simulink model "part2"  (R2019b)
settings: Solver=FixedStepAuto  StartTime=0.0  StopTime=1000  FixedStep=0.1  RelTol=1e-3
values from neighbouring files (symbols this model uses):
  A_w = [zeros(3) eye(3) ... (first row only)    [initObs.m]
  B_pseudo = inv(W)*B_u'*inv(B_u*inv(W)*B_u' + epsilon.*eye(3))    [init_thrustAloc.m]
  C_w = [zeros(3) eye(3)]    [initObs.m]
  constant_dp = 0    [pick_sp.m]
  corner_test = 0    [pick_sp.m]
  corners = [0,0,0;50,0,0;50,-50,0;50,-50,-pi/4;0,-50,-pi/4;0,0,0]    [pick_sp.m]
  curr_mean_dir = curr_mean_dir + 10    (= 10)    [capabilitytest.m]    (also in pick_sp.m = 270)
  curr_mean_vel = 0.2    [pick_sp.m]
  D = diag([2.6486e+05,8.8164e+05,3.3774e+08])    [init.m]    (also in initObs.m = [2.648*10^5 0 0)
  Delta_stack = zeros(15,3,360)    [init_kalman.m]
  Gamma_stack = zeros(15,6,360)    [init_kalman.m]
  H = [Cw, eye(3),zeros(3,6)]    [init_kalman.m]
  K1 = [-2*(zeta_ni_nop - zeta_i_nop)*(omega_ci_nop/omega_p)*eye(3) ... (first row only)    [initObs.m]
  K2 = diag([omega_ci_nop omega_ci_nop omega_ci_nop])    [initObs.m]
  K3 = 0.1*K4    [initObs.m]
  K4 = diag([0.1 0.1 0.01])    [initObs.m]
  Kd = [1e+07,1e+07,2.01e+08]    [tune.m]
  Ki = [2e+02,2e+02,1e+02]    [tune.m]
  Kp = [1e+05,5e+05,1e+07]    [tune.m]
  M = [6.8177e+06,0,0;0,7.8784e+06,-2.5955e+06;0,-2.5955e+06,3.57e+09]    [init.m]    (also in initObs.m = [ 6.8177*10^6 0 0)
  observer_on = 1    [pick_sp.m]
  Phi_stack = zeros(15,15,360)    [init_kalman.m]
  Q = diag([Q1 Q2])    [init_kalman.m]
  R_KF = diag([0 0 0])    [init_kalman.m]
  ref_model_on = 1    [pick_sp.m]
  setpoint = [0,0,0]    [pick_sp.m]
  T_b = diag([1000 1000 1000])    [initObs.m]
  thrusters =     [thrusters_sup.mat]
  use_kalman = 1    [pick_sp.m]
  vessel =     [thrusters_sup.mat]
  w_n = [0.08,0.04,0.03]    [tune.m]
  wave_mean_dir = wave_mean_dir + (10*pi/180)    (= 0.174532925199)    [capabilitytest.m]    (also in pick_sp.m = 225)
  wave_peak_T = 13    [pick_sp.m]
  wind_mean_dir = wind_mean_dir + (10*pi/180)    (= 0.174532925199)    [capabilitytest.m]    (also in pick_sp.m = 180)
  wind_mean_vel = 15    [pick_sp.m]
  zeta = 1    [tune.m]
undefined symbols (not defined in the file or in its folder): Hoerner, magnitude
libraries: marine_gnc x13, simulink x4, cstblocks x4, marine_hydro x2
(part 1 of 2)
settings Model: Creator=jonbjor  LastModifiedBy=Elias
settings DataIOCC: ReturnWorkspaceOutputs=off
settings DebuggingCC: ArithmeticOperatorsInVariantConditions=warning
settings SFSimCC: SimUseLocalCustomCode=off  CustomCodeUndefinedFunction=UseInterfaceOnly
settings RTWCC: RTWUseLocalCustomCode=off

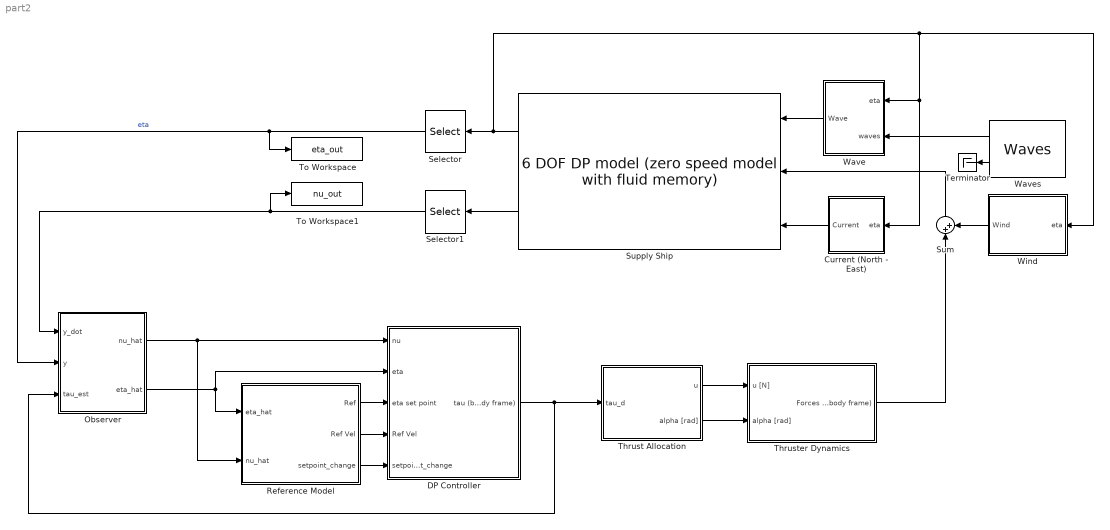
== system part2 ==
  Current (North - East) : Subsystem
  DP Controller : Subsystem
  Observer : Subsystem
  Reference Model : Subsystem
  Selector : Selector  InputPortWidth=6  IndexOptions=Index vector (dialog)  Indices=[1 2 6]  OutputSizes=1
  Selector1 : Selector  InputPortWidth=6  IndexOptions=Index vector (dialog)  Indices=[1 2 6]  OutputSizes=1
  Sum : Sum  Inputs=|++
  Supply Ship : marine_hydro/Hydro Library/6 DOF DP model  (zero speed model with fluid memory)  ABC=vesselABC  rho=1025  Axc=0.9*vessel.main.T*vessel.main.B  Ayc=0.9*vessel.main.T*vessel.main.Lpp  CX=1  CY_2D=Hoerner(vessel.main.B,vessel.main.T)  Bv=vessel.Bv  mask(6 DOF zero speed model){}
      link override "Integrator1 ": InitialCondition=nu0
      link override Integrator2: InitialCondition=eta0
      settings: SourceProductName=MSS Hydro
      mask Display:
      | image('supply.jpg');
      | color('white'); port_label('output', 1, 'eta')
      | color('white'); port_label('output', 2, 'nu')
      | color('white'); port_label('input', 1, 'tau_wave')
      | color('white'); port_label('input', 2, 'tau')
      | color('white'); port_label('input', 3, 'nu_c')
  Terminator : Terminator
  Thrust Allocation : Subsystem
  Thruster Dynamics : Subsystem  mask{thrusterfault=off}
      mask prompts: thrusterfault "Fault on thruster #2 and #5?"
  To Workspace : ToWorkspace  VariableName=eta_out  SampleTime=-1
  To Workspace1 : ToWorkspace  VariableName=nu_out  SampleTime=-1
  Wave : Subsystem  mask{waveforces=off}
      mask prompts: waveforces "Waveforces enabled"
  Waves : marine_gnc/Environment/Waves/Waves  spectrum_type=ITTC  disp_flag=on  plot_spectrum=off  plot_realization=off  hs=wave_height  omega_peak=2*pi/wave_peak_T  psi_mean=wave_mean_dir*pi/180  gamma=-1  spread=2  depth=inf  nfreq=100  ndir=10  energylim=0.005  freq_cutoff=3  dir_cutoff=0  rand_seed=1234  rand_freq=off  rand_dir=off  Zeta_a=0  Omega=0  Phase=0  Wavenum=0  Psi=0
      settings: SourceProductName=MSS GNC
  Wind : Subsystem
  wires:
  Supply Ship/2 -> Selector1/1
  Supply Ship/1 -> Wind/1("eta "), Current (North - East)/1(eta), Wave/1(eta), Selector/1
  Waves/1 -> Wave/2(waves)
  Waves/2 -> Terminator/1
  Selector1/1 -> To Workspace1/1, Observer/1(y_dot)
  Observer/1(nu_hat) -> Reference Model/2(nu_hat), DP Controller/1(nu)
  Sum/1 -> Supply Ship/2
  Selector/1 -> To Workspace/1, Observer/2(y)  "eta"
  Reference Model/1("Ref ") -> DP Controller/3(eta set point)
  Observer/2(eta_hat) -> Reference Model/1(eta_hat), DP Controller/2(eta)
  Reference Model/2("Ref Vel ") -> DP Controller/4("Ref Vel ")
  Current (North - East)/1(Current) -> Supply Ship/3
  Wave/1(Wave) -> Supply Ship/1
  Wind/1(Wind) -> Sum/2
  Thrust Allocation/2(alpha [rad]) -> Thruster Dynamics/2(alpha [rad])
  Thruster Dynamics/1("Forces (body frame) ") -> Sum/1
  Thrust Allocation/1("u ") -> Thruster Dynamics/1(u [N])
  DP Controller/1(tau (body frame)) -> Thrust Allocation/1(tau_d), Observer/3(tau_est)
  Reference Model/3(setpoint_change) -> DP Controller/5(setpoint_change)

== system part2/Current (North - East) ==
  eta : Inport
  "Angle variation " : Subsystem
  Constant : Constant  Value=curr_mean_vel
  Constant2 : Constant  Value=curr_mean_dir
  North-East current : marine_gnc/Environment/Current/North-East current  SystemSampleTime=-1  Latency=0  AutoFrameSizeCalculation=off
      settings: SourceProductName=MSS GNC
  "RFC " : Subsystem
  Velocity variation : Subsystem
  Current : Outport  VectorParamsAs1DForOutWhenUnconnected=off
  wires:
  Constant/1 -> Velocity variation/1(Mean Vel)
  eta/1 -> "RFC "/1(eta)
  North-East current/1 -> "RFC "/2("Current (NED) ")
  "RFC "/1("Current (Body) ") -> Current/1
  Constant2/1 -> "Angle variation "/1(Mean Dir)
  "Angle variation "/1(Current Dir) -> North-East current/1
  Velocity variation/1(Current Vel) -> North-East current/2

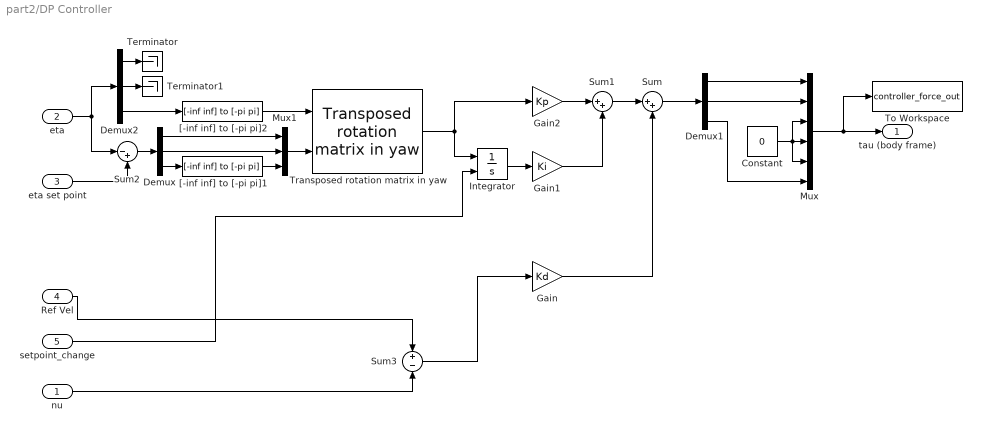
== system part2/DP Controller ==
  nu : Inport  PortDimensions=3
  eta : Inport  Port=2  PortDimensions=3
  eta set point : Inport  Port=3
  "Ref Vel " : Inport  Port=4
  setpoint_change : Inport  Port=5
  Constant : Constant  Value=0
  Demux : Demux  Outputs=3
  Demux1 : Demux  Outputs=3
  Demux2 : Demux  Outputs=3
  Gain : Gain  Gain=Kd
  Gain1 : Gain  Gain=Ki
  Gain2 : Gain  Gain=Kp
  Integrator : Integrator  ExternalReset=level hold
  Mux : Mux  Inputs=6
  Mux1 : Mux  Inputs=3
  Sum : Sum  Inputs=|++
  Sum1 : Sum  Inputs=|++
  Sum2 : Sum  Inputs=|-+
  Sum3 : Sum  Inputs=+|-
  Terminator : Terminator
  Terminator1 : Terminator
  To Workspace : ToWorkspace  VariableName=controller_force_out  SampleTime=-1
  Transposed rotation matrix in yaw : marine_gnc/Models/ Kinematics/Transposed rotation  matrix in yaw
      settings: SourceProductName=MSS GNC
  "[-inf inf] to [-pi pi]1" : marine_gnc/Utilities/Math Operations/[-inf inf] to [-pi pi]
      settings: SourceProductName=MSS GNC
  "[-inf inf] to [-pi pi]2" : marine_gnc/Utilities/Math Operations/[-inf inf] to [-pi pi]
      settings: SourceProductName=MSS GNC
  tau (body frame) : Outport  VectorParamsAs1DForOutWhenUnconnected=off
  wires:
  Demux2/2 -> Terminator1/1
  Demux/3 -> "[-inf inf] to [-pi pi]1"/1
  Sum2/1 -> Demux/1
  Demux1/1 -> Mux/1
  "[-inf inf] to [-pi pi]2"/1 -> Transposed rotation matrix in yaw/1
  "[-inf inf] to [-pi pi]1"/1 -> Mux1/3
  Mux/1 -> To Workspace/1, tau (body frame)/1
  Demux/1 -> Mux1/1
  Demux1/2 -> Mux/2
  Demux2/3 -> "[-inf inf] to [-pi pi]2"/1
  Constant/1 -> Mux/5, Mux/3, Mux/4
  Mux1/1 -> Transposed rotation matrix in yaw/2
  Integrator/1 -> Gain1/1
  eta/1 -> Demux2/1, Sum2/1
  Gain2/1 -> Sum1/1
  Gain1/1 -> Sum1/2
  Demux2/1 -> Terminator/1
  Demux/2 -> Mux1/2
  Demux1/3 -> Mux/6
  Sum/1 -> Demux1/1
  Sum1/1 -> Sum/1
  Gain/1 -> Sum/2
  eta set point/1 -> Sum2/2
  Transposed rotation matrix in yaw/1 -> Integrator/1, Gain2/1
  nu/1 -> Sum3/2
  Sum3/1 -> Gain/1
  "Ref Vel "/1 -> Sum3/1
  setpoint_change/1 -> Integrator/2

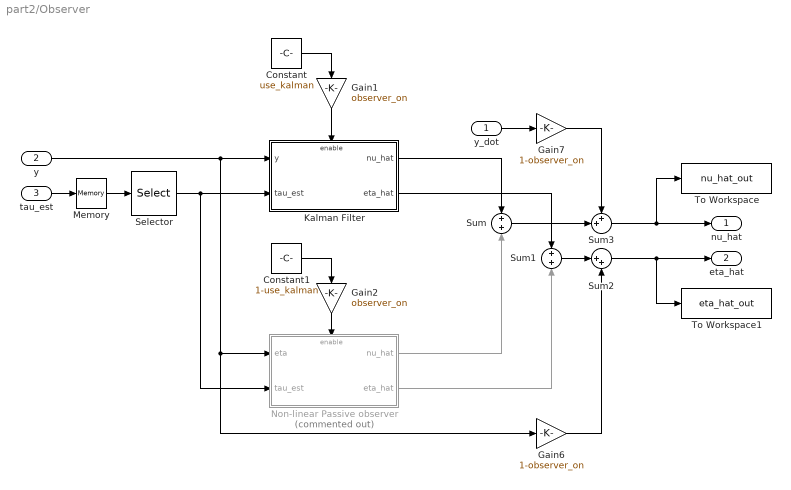
== system part2/Observer ==
  y_dot : Inport
  y : Inport  Port=2
  tau_est : Inport  Port=3
  Constant : Constant  Value=use_kalman
  Constant1 : Constant  Value=1-use_kalman
  Gain1 : Gain  Gain=observer_on
  Gain2 : Gain  Gain=observer_on
  Gain6 : Gain  Gain=1-observer_on
  Gain7 : Gain  Gain=1-observer_on
  "Kalman Filter " : Subsystem
  Memory : Memory
  Non-linear Passive observer : Subsystem  Commented=on
  Selector : Selector  InputPortWidth=6  IndexOptions=Index vector (dialog)  Indices=[1 2 6]  OutputSizes=1
  Sum : Sum  Inputs=+|+
  Sum1 : Sum  Inputs=+|+
  Sum2 : Sum  Inputs=|++
  Sum3 : Sum  Inputs=++|
  To Workspace : ToWorkspace  VariableName=nu_hat_out  SampleTime=-1
  To Workspace1 : ToWorkspace  VariableName=eta_hat_out  SampleTime=-1
  nu_hat : Outport  VectorParamsAs1DForOutWhenUnconnected=off
  eta_hat : Outport  Port=2  VectorParamsAs1DForOutWhenUnconnected=off
  wires:
  Gain6/1 -> Sum2/2
  y_dot/1 -> Gain7/1
  Gain7/1 -> Sum3/1
  Sum3/1 -> To Workspace/1, nu_hat/1
  Sum2/1 -> To Workspace1/1, eta_hat/1
  y/1 -> "Kalman Filter "/1(y), Non-linear Passive observer/1(eta), Gain6/1
  tau_est/1 -> Memory/1
  "Kalman Filter "/1(nu_hat) -> Sum/1
  "Kalman Filter "/2(eta_hat) -> Sum1/1
  Non-linear Passive observer/1(nu_hat) -> Sum/2
  Non-linear Passive observer/2(eta_hat) -> Sum1/2
  Sum/1 -> Sum3/2
  Sum1/1 -> Sum2/1
  Constant/1 -> Gain1/1
  Gain1/1 -> "Kalman Filter "/Enable
  Constant1/1 -> Gain2/1
  Gain2/1 -> Non-linear Passive observer/Enable
  Selector/1 -> Non-linear Passive observer/2(tau_est), "Kalman Filter "/2(tau_est)
  Memory/1 -> Selector/1

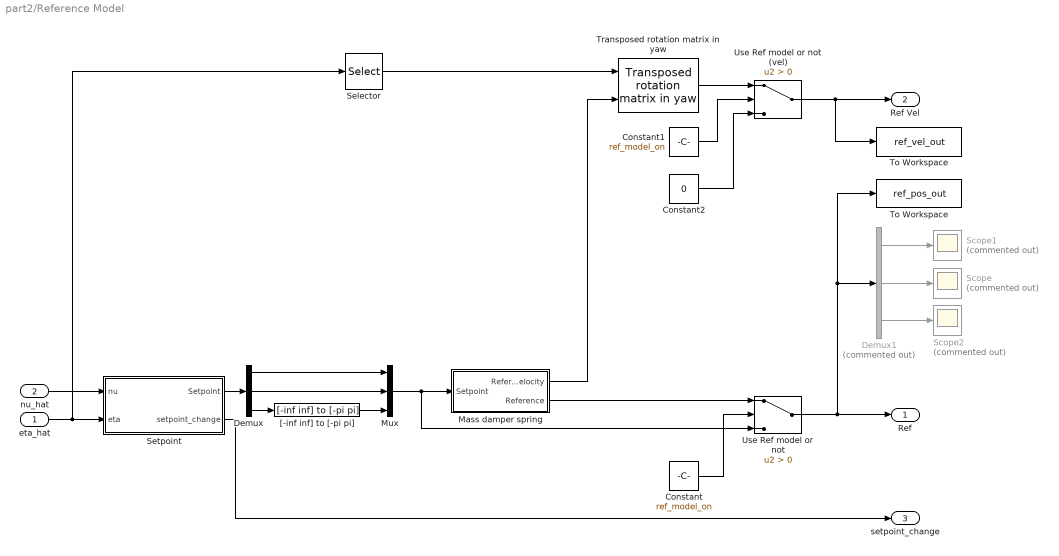
== system part2/Reference Model ==
  eta_hat : Inport
  nu_hat : Inport  Port=2
  Constant : Constant  Value=ref_model_on
  Constant1 : Constant  Value=ref_model_on
  Constant2 : Constant  Value=0
  Demux : Demux  Outputs=3
  Demux1 : Demux  Commented=on  Outputs=3
  Mass damper spring : Subsystem
  Mux : Mux  Inputs=3
  Scope : Scope  Commented=on
  Scope1 : Scope  Commented=on
  Scope2 : Scope  Commented=on
  Selector : Selector  InputPortWidth=3  IndexOptions=Index vector (dialog)  Indices=[3]  OutputSizes=1
  "Setpoint " : Subsystem
  To Workspace : ToWorkspace  VariableName=ref_vel_out  SampleTime=-1
  "To Workspace " : ToWorkspace  VariableName=ref_pos_out  SampleTime=-1
  Transposed rotation matrix in yaw : marine_gnc/Models/ Kinematics/Transposed rotation  matrix in yaw
      settings: SourceProductName=MSS GNC
  Use Ref model or not : Switch  Criteria=u2 > Threshold
  "Use Ref model or not (vel) " : Switch  Criteria=u2 > Threshold
  "[-inf inf] to [-pi pi]" : marine_gnc/Utilities/Math Operations/[-inf inf] to [-pi pi]
      settings: SourceProductName=MSS GNC
  "Ref " : Outport  VectorParamsAs1DForOutWhenUnconnected=off
  "Ref Vel " : Outport  Port=2  VectorParamsAs1DForOutWhenUnconnected=off
  setpoint_change : Outport  Port=3
  wires:
  Mass damper spring/2("Reference ") -> Use Ref model or not/1
  Use Ref model or not/1 -> "Ref "/1, "To Workspace "/1, Demux1/1
  Mass damper spring/1("Reference Velocity ") -> Transposed rotation matrix in yaw/2
  Mux/1 -> Use Ref model or not/3, Mass damper spring/1("Setpoint ")
  Demux1/2 -> Scope/1
  Demux/3 -> "[-inf inf] to [-pi pi]"/1
  "[-inf inf] to [-pi pi]"/1 -> Mux/3
  Demux1/3 -> Scope2/1
  Demux1/1 -> Scope1/1
  "Setpoint "/1("Setpoint ") -> Demux/1
  Demux/1 -> Mux/1
  Demux/2 -> Mux/2
  Selector/1 -> Transposed rotation matrix in yaw/1
  eta_hat/1 -> Selector/1, "Setpoint "/2("eta ")
  nu_hat/1 -> "Setpoint "/1(nu)
  Constant/1 -> Use Ref model or not/2
  Transposed rotation matrix in yaw/1 -> "Use Ref model or not (vel) "/1
  Constant1/1 -> "Use Ref model or not (vel) "/2
  Constant2/1 -> "Use Ref model or not (vel) "/3
  "Use Ref model or not (vel) "/1 -> To Workspace/1, "Ref Vel "/1
  "Setpoint "/2(setpoint_change) -> setpoint_change/1

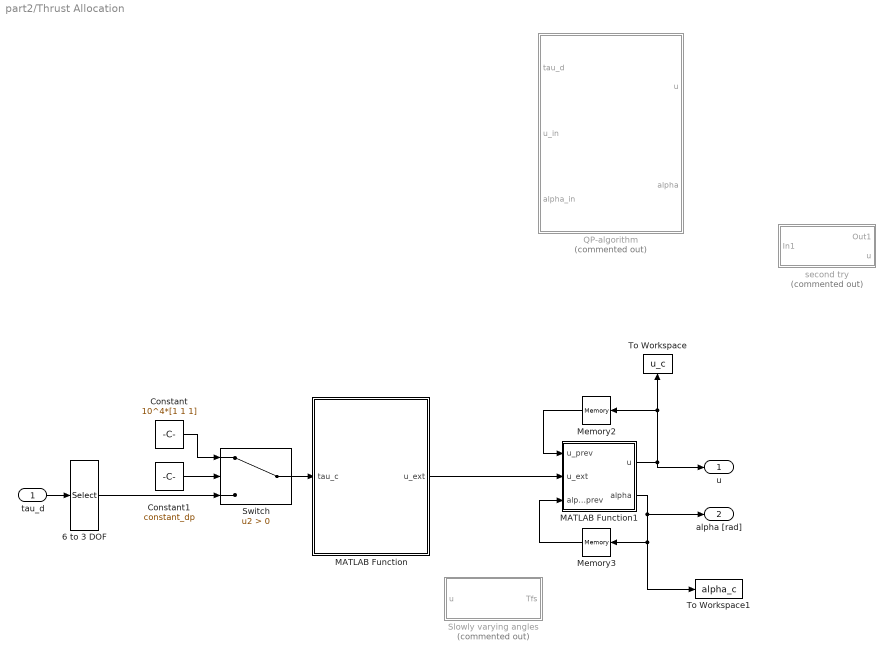
== system part2/Thrust Allocation ==
  tau_d : Inport
  6 to 3 DOF : Selector  InputPortWidth=6  IndexOptions=Index vector (dialog)  Indices=[1 2 6]  OutputSizes=1
  Constant : Constant  Value=10^4*[1 1 1]
  Constant1 : Constant  Value=constant_dp
  MATLAB Function : MATLAB Function  TreatAsAtomicUnit=on
  MATLAB Function1 : MATLAB Function  TreatAsAtomicUnit=on
  Memory2 : Memory
  Memory3 : Memory
  QP-algorithm : MATLAB Function  Commented=on  TreatAsAtomicUnit=on
  Slowly varying angles : Subsystem  Commented=on
  Switch : Switch  Criteria=u2 > Threshold
  To Workspace : ToWorkspace  VariableName=u_c  SampleTime=-1
  To Workspace1 : ToWorkspace  VariableName=alpha_c  SampleTime=-1
  second try : Subsystem  Commented=on
  "u " : Outport  VectorParamsAs1DForOutWhenUnconnected=off
  alpha [rad] : Outport  Port=2  VectorParamsAs1DForOutWhenUnconnected=off
  wires:
  tau_d/1 -> 6 to 3 DOF/1
  6 to 3 DOF/1 -> Switch/3
  MATLAB Function1/2(alpha) -> To Workspace1/1, Memory3/1, alpha [rad]/1
  MATLAB Function1/1(u) -> "u "/1, To Workspace/1, Memory2/1
  Memory3/1 -> MATLAB Function1/3(alpha_prev)
  Memory2/1 -> MATLAB Function1/1(u_prev)
  MATLAB Function/1(u_ext) -> MATLAB Function1/2(u_ext)
  Constant/1 -> Switch/1
  Switch/1 -> MATLAB Function/1(tau_c)
  Constant1/1 -> Switch/2

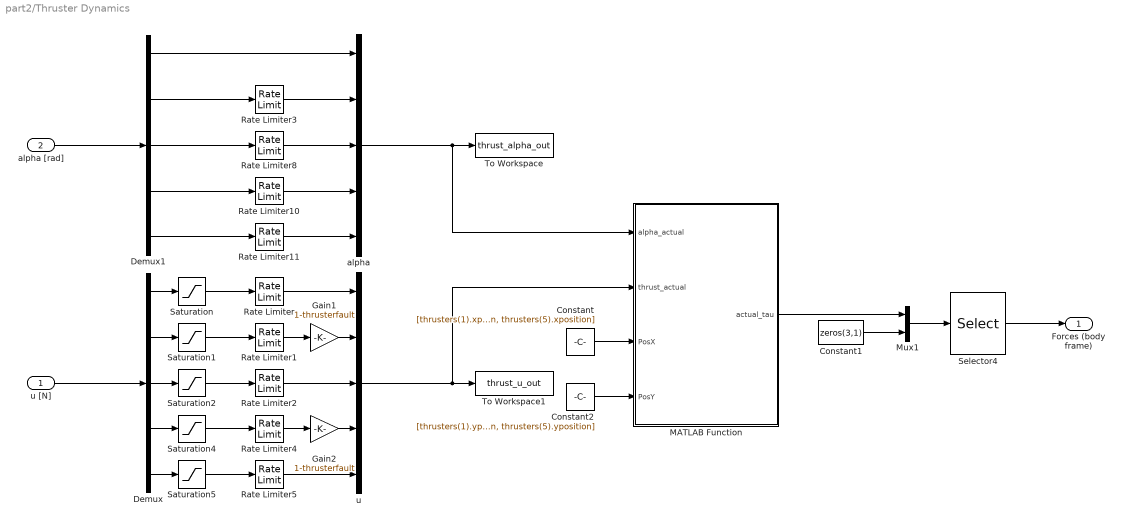
== system part2/Thruster Dynamics ==
  u [N] : Inport
  alpha [rad] : Inport  Port=2
  Constant : Constant  Value=[thrusters(1).xposition, thrusters(2).xposition, thrusters(3).xposition, thrusters(4).xposition, thrusters(5).xposition]
  Constant1 : Constant  Value=zeros(3,1)
  Constant2 : Constant  Value=[thrusters(1).yposition, thrusters(2).yposition, thrusters(3).yposition, thrusters(4).yposition, thrusters(5).yposition]
  Demux : Demux  Outputs=5
  Demux1 : Demux  Outputs=5
  Gain1 : Gain  Gain=1-thrusterfault
  Gain2 : Gain  Gain=1-thrusterfault
  MATLAB Function : MATLAB Function  TreatAsAtomicUnit=on
  Mux1 : Mux  Inputs=2
  Rate Limiter : RateLimiter  RisingSlewLimit=thrusters(1).rate  FallingSlewLimit=-thrusters(1).rate  SampleTimeMode=inherited
  Rate Limiter1 : RateLimiter  RisingSlewLimit=thrusters(2).rate  FallingSlewLimit=-thrusters(2).rate  SampleTimeMode=inherited
  Rate Limiter10 : RateLimiter  RisingSlewLimit=thrusters(4).rotationspeed  FallingSlewLimit=-thrusters(4).rotationspeed  SampleTimeMode=inherited
  Rate Limiter11 : RateLimiter  RisingSlewLimit=thrusters(5).rotationspeed  FallingSlewLimit=-thrusters(5).rotationspeed  SampleTimeMode=inherited
  Rate Limiter2 : RateLimiter  RisingSlewLimit=thrusters(3).rate  FallingSlewLimit=-thrusters(3).rate  SampleTimeMode=inherited
  Rate Limiter3 : RateLimiter  RisingSlewLimit=thrusters(2).rotationspeed  FallingSlewLimit=-thrusters(2).rotationspeed  SampleTimeMode=inherited
  Rate Limiter4 : RateLimiter  RisingSlewLimit=thrusters(4).rate  FallingSlewLimit=-thrusters(4).rate  SampleTimeMode=inherited
  Rate Limiter5 : RateLimiter  RisingSlewLimit=thrusters(5).rate  FallingSlewLimit=-thrusters(5).rate  SampleTimeMode=inherited
  Rate Limiter8 : RateLimiter  RisingSlewLimit=thrusters(3).rotationspeed  FallingSlewLimit=-thrusters(3).rotationspeed  SampleTimeMode=inherited
  Saturation : Saturate  UpperLimit=thrusters(1).thrust  LowerLimit=-thrusters(1).thrust
  Saturation1 : Saturate  UpperLimit=thrusters(2).thrust  LowerLimit=-thrusters(2).thrust
  Saturation2 : Saturate  UpperLimit=thrusters(3).thrust  LowerLimit=-thrusters(3).thrust
  Saturation4 : Saturate  UpperLimit=thrusters(4).thrust  LowerLimit=-thrusters(4).thrust
  Saturation5 : Saturate  UpperLimit=thrusters(5).thrust  LowerLimit=-thrusters(5).thrust
  Selector4 : Selector  InputPortWidth=6  IndexOptions=Index vector (dialog)  Indices=[1 2 4 5 6 3]  OutputSizes=1
  To Workspace : ToWorkspace  VariableName=thrust_alpha_out  SampleTime=-1
  To Workspace1 : ToWorkspace  VariableName=thrust_u_out  SampleTime=-1
  alpha : Mux  Inputs=5
  u : Mux  Inputs=5
  "Forces (body frame) " : Outport  VectorParamsAs1DForOutWhenUnconnected=off
  wires:
  Rate Limiter2/1 -> u/3
  Saturation/1 -> Rate Limiter/1
  Mux1/1 -> Selector4/1
  Constant1/1 -> Mux1/2
  Saturation4/1 -> Rate Limiter4/1
  Demux/2 -> Saturation1/1
  Saturation1/1 -> Rate Limiter1/1
  Demux/1 -> Saturation/1
  Demux/3 -> Saturation2/1
  Saturation2/1 -> Rate Limiter2/1
  Selector4/1 -> "Forces (body frame) "/1
  Gain1/1 -> u/2
  Rate Limiter1/1 -> Gain1/1
  Rate Limiter/1 -> u/1
  Rate Limiter4/1 -> Gain2/1
  Saturation5/1 -> Rate Limiter5/1
  Rate Limiter8/1 -> alpha/3
  u [N]/1 -> Demux/1
  alpha [rad]/1 -> Demux1/1
  Constant/1 -> MATLAB Function/3(PosX)
  Constant2/1 -> MATLAB Function/4(PosY)
  u/1 -> To Workspace1/1, MATLAB Function/2(thrust_actual)
  alpha/1 -> To Workspace/1, MATLAB Function/1(alpha_actual)
  MATLAB Function/1(actual_tau) -> Mux1/1
  Demux1/3 -> Rate Limiter8/1
  Rate Limiter10/1 -> alpha/4
  Demux1/4 -> Rate Limiter10/1
  Demux1/5 -> Rate Limiter11/1
  Rate Limiter11/1 -> alpha/5
  Demux1/2 -> Rate Limiter3/1
  Demux1/1 -> alpha/1
  Gain2/1 -> u/4
  Demux/4 -> Saturation4/1
  Demux/5 -> Saturation5/1
  Rate Limiter5/1 -> u/5
  Rate Limiter3/1 -> alpha/2

== system part2/Wave ==
  eta : Inport
  waves : Inport  Port=2
  Gain : Gain  Gain=waveforces
  Sum : Sum
  To Workspace : ToWorkspace  VariableName=wave_force  SampleTime=-1
  Wave loads (U=0) : marine_hydro/Hydro Library/Wave loads (U=0)  SystemSampleTime=-1  Latency=0  AutoFrameSizeCalculation=off
      settings: SourceProductName=MSS Hydro
  Wave : Outport  VectorParamsAs1DForOutWhenUnconnected=off
  wires:
  eta/1 -> Wave loads (U=0)/1
  waves/1 -> Wave loads (U=0)/2
  Sum/1 -> Gain/1
  Wave loads (U=0)/1 -> Sum/1
  Wave loads (U=0)/2 -> Sum/2
  Gain/1 -> To Workspace/1, Wave/1

== system part2/Wind ==
  "eta " : Inport
  Convert angle to index in wind_coeff : MATLAB Function  TreatAsAtomicUnit=on
  Direct Lookup Table (n-D) : LookupNDDirect  InputsSelectThisObjectFromTable=Vector  Table=wind_coeff_matrix'
  Product : Product
  Selector : Selector  InputPortWidth=6  IndexOptions=Index vector (dialog)  Indices=[6]  OutputSizes=1
  Square : Math  Operator=magnitude^2  SignedPower=off  SaturateOnIntegerOverflow=on
  Sum : Sum  Inputs=|+-
  Wind mean + Gust + Slowly Varying : Subsystem  mask(Wind){page=1, Par_Wind_slowlyvar=on, Par_Wind_gust=on, Par_Wind_V=wind_mean_vel, Par_Wind_angle=wind_mean_dir, Par_Wind_spectrum_type=2, Par_Wind_z=10, Par_Wind_sample_time=1, Par_Wind_speed_T=10, Par_Wind_angle_T=10, Par_Wind_speed_noise_pow=0.005, Par_Wind_angle_noise_pow=0.005, Par_Wind_speed_rand_max=0.01, Par_Wind_angle_rand_max=pi/36, Par_Wind_speed_seed=123, Par_Wind_angle_seed=321, Par_Wind_phase_seed=1337, Par_Wind_kappa_H=0.0026, Par_Wind_L=1800, Par_Wind_minfreq=1E-4, Par_Wind_maxfreq=0.1, Par_Wind_nfreq=100}
      mask prompts: Par_Wind_slowlyvar "Include slowly-varing wind velocity and direction"; Par_Wind_gust "Include wind gust"; Par_Wind_V "Mean wind velocity [m/s]"; Par_Wind_angle "Mean wind angle [rad]"; Par_Wind_spectrum_type "Wind gust spectrum type"; Par_Wind_z "Height over water surface [m (for NORSOK wind spectrum)]"; Par_Wind_sample_time "Wind sample time [s]"; Par_Wind_speed_T "Wind speed time constant [s]"; Par_Wind_angle_T "Wind angle time constant [s]"; Par_Wind_speed_noise_pow "Wind speed noise power"; Par_Wind_angle_noise_pow "Wind angle noise power"; Par_Wind_speed_rand_max "Wind speed saturation [m/s] (max random variation about mean)"; Par_Wind_angle_rand_max "Wind angle saturation [rad] (max random variation about mean)"; Par_Wind_speed_seed "Wind speed random seed"; Par_Wind_angle_seed "Wind angle random seed"; Par_Wind_phase_seed "Wind gust phase seed"; Par_Wind_kappa_H "Sea surface drag coefficient for Harris wind spectrum (0.0026)"; Par_Wind_L "Scaling length for Harris wind spectrum (1800)"; Par_Wind_minfreq "Minimum frequency in gust [Hz] (1E-4)"; Par_Wind_maxfreq "Maximum frequency in gust [Hz] (0.1)"; Par_Wind_nfreq "Number of frequency components"
      mask help:
      | Generates wind speed and direction based on the mean angle and mean wind speed at 10 meters height. The total velocity is composed of a slowly-varying mean superposed with gusts based on a chosen wind spectrum. The direction is slowly-varying based on a random process.
      |
      | The wind spectrum types are:
      |
      | 1) Harris         (based on measurements over land)
      | 2) NORSOK   (based on measurements from the North Sea)
      mask Help:
      | <b>Part of the Marine Systems Simulator: MSS</b><p>Generate wind speed and direction based on the mean angle and mean wind
      | speed at 10 meters height. The total velocity is composed of a slowly-varying
      | mean superposed with gusts based on a chosen wind spectrum. The direction is
      | slowly-varying based on a random process.<br>
      | <br>
      | The wind spectrum types are:<br>
      | <br>
      | 1) Harris (based on measurements over land)<br>
      | 2) NORSOK (based on measurements from the North Sea)</p>
      | <p>The wind gust from the Harris spectrum is uniform over the height, whereas
      | the wind gust from the NORSOK spectrum varies with the height.</p>
      | <p>The random variation of the mean speed and angle can be limited by two saturation
      | parameters, which define the maximum random deviation from the mean value.<p><b>Outputs:
      | </b> </p>
      | <p>angle: [rad] Wind angle in the n-frame<br>
      | speed: [m/s] Wind velocity in the n-frame<p>
      | <b>Copyright NTNU 2005</b></p>
      | <p><b>Author:</b> Oyvind N. Smogeli, 2005-05-03</p>
      mask TypeOptions page: 1 | 2
      mask Callback page: MSS_mask_page(12);
      mask TypeOptions Par_Wind_spectrum_type: 1 | 2
  "[-inf inf] to [-pi pi]1" : marine_gnc/Utilities/Math Operations/[-inf inf] to [-pi pi]
      settings: SourceProductName=MSS GNC
  Wind : Outport  VectorParamsAs1DForOutWhenUnconnected=off
  wires:
  Wind mean + Gust + Slowly Varying/2(speed) -> Square/1
  Square/1 -> Product/2
  Product/1 -> Wind/1
  "eta "/1 -> Selector/1
  Selector/1 -> Sum/1
  Wind mean + Gust + Slowly Varying/1(angle) -> Sum/2
  Sum/1 -> "[-inf inf] to [-pi pi]1"/1
  "[-inf inf] to [-pi pi]1"/1 -> Convert angle to index in wind_coeff/1(ang)
  Convert angle to index in wind_coeff/1(index) -> Direct Lookup Table (n-D)/1
  Direct Lookup Table (n-D)/1 -> Product/1

== system part2/Current (North - East)/Angle variation  ==
  Mean Dir : Inport
  Band-Limited White Noise : simulink/Sources/Band-Limited White Noise  Cov=0.005  Ts=1  seed=[23341]
  Gain : Gain  Gain=0.001
  Integrator : Integrator
  Saturation : Saturate  UpperLimit=5  LowerLimit=-5
  Sum : Sum  Inputs=|+-
  Sum1 : Sum  Inputs=++|
  Current Dir : Outport
  wires:
  Band-Limited White Noise/1 -> Sum/1
  Sum/1 -> Integrator/1
  Gain/1 -> Sum/2
  Sum1/1 -> Current Dir/1
  Mean Dir/1 -> Sum1/1
  Integrator/1 -> Saturation/1, Gain/1
  Saturation/1 -> Sum1/2

== system part2/Current (North - East)/RFC  ==
  eta : Inport
  "Current (NED) " : Inport  Port=2
  Constant : Constant  Value=0
  Demux : Demux  Outputs=6
  Demux2 : Demux  Outputs=3
  Mux : Mux  Inputs=3
  Mux1 : Mux  Inputs=6
  Selector : Selector  InputPortWidth=6  IndexOptions=Index vector (dialog)  Indices=[6]  OutputSizes=1
  Terminator : Terminator
  Terminator1 : Terminator
  Terminator2 : Terminator
  Transposed rotation matrix in yaw : marine_gnc/Models/ Kinematics/Transposed rotation  matrix in yaw
      settings: SourceProductName=MSS GNC
  "Current (Body) " : Outport
  wires:
  eta/1 -> Selector/1
  Selector/1 -> Transposed rotation matrix in yaw/1
  Demux/3 -> Mux/3
  Demux/2 -> Mux/2
  Demux/1 -> Mux/1
  Mux/1 -> Transposed rotation matrix in yaw/2
  Mux1/1 -> "Current (Body) "/1
  Transposed rotation matrix in yaw/1 -> Demux2/1
  Demux2/3 -> Mux1/6
  Demux2/1 -> Mux1/1
  Constant/1 -> Mux1/5, Mux1/3, Mux1/4
  "Current (NED) "/1 -> Demux/1
  Demux/4 -> Terminator/1
  Demux/5 -> Terminator1/1
  Demux/6 -> Terminator2/1
  Demux2/2 -> Mux1/2

== system part2/Current (North - East)/Velocity variation ==
  Mean Vel : Inport
  Band-Limited White Noise : simulink/Sources/Band-Limited White Noise  Cov=0.005  Ts=1  seed=[13371]
  Gain : Gain  Gain=0.001
  Integrator : Integrator
  Saturation : Saturate  UpperLimit=0.002  LowerLimit=-0.002
  Sum : Sum  Inputs=|+-
  Sum1 : Sum  Inputs=++|
  Current Vel : Outport
  wires:
  Band-Limited White Noise/1 -> Sum/1
  Sum/1 -> Integrator/1
  Gain/1 -> Sum/2
  Sum1/1 -> Current Vel/1
  Mean Vel/1 -> Sum1/1
  Integrator/1 -> Saturation/1, Gain/1
  Saturation/1 -> Sum1/2

== system part2/Observer/Kalman Filter  ==
  y : Inport
  tau_est : Inport  Port=2
  Enable : EnablePort  StatesWhenEnabling=reset
  Extended Kalman Filter : Subsystem
  nu_hat : Outport
  eta_hat : Outport  Port=2
  wires:
  tau_est/1 -> Extended Kalman Filter/2(u)
  y/1 -> Extended Kalman Filter/1(y)
  Extended Kalman Filter/2(eta_hat) -> eta_hat/1
  Extended Kalman Filter/1(nu_hat) -> nu_hat/1

== system part2/Observer/Non-linear Passive observer ==
  eta : Inport
  tau_est : Inport  Port=2
  Enable : EnablePort  StatesWhenEnabling=reset
  Subsystem : Subsystem
  nu_hat : Outport
  eta_hat : Outport  Port=2
  wires:
  Subsystem/1(nu_hat) -> nu_hat/1
  Subsystem/2(eta_hat_total) -> eta_hat/1
  eta/1 -> Subsystem/1(eta)
  tau_est/1 -> Subsystem/2(tau_est)

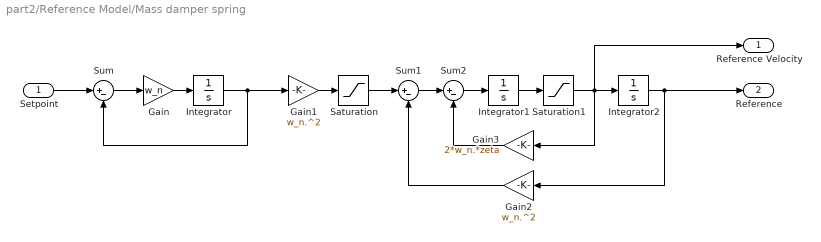
== system part2/Reference Model/Mass damper spring ==
  "Setpoint " : Inport
  Gain : Gain  Gain=w_n
  Gain1 : Gain  Gain=w_n.^2
  Gain2 : Gain  Gain=w_n.^2
  Gain3 : Gain  Gain=2*w_n.*zeta
  Integrator : Integrator
  Integrator1 : Integrator
  Integrator2 : Integrator
  Saturation : Saturate  UpperLimit=25  LowerLimit=-25
  Saturation1 : Saturate  UpperLimit=25  LowerLimit=-25
  Sum : Sum  Inputs=|+-
  Sum1 : Sum  Inputs=|+-
  Sum2 : Sum  Inputs=|+-
  "Reference Velocity " : Outport
  "Reference " : Outport  Port=2
  wires:
  Gain1/1 -> Saturation/1
  Saturation/1 -> Sum1/1
  Saturation1/1 -> "Reference Velocity "/1, Gain3/1, Integrator2/1
  Gain/1 -> Integrator/1
  Sum2/1 -> Integrator1/1
  Integrator1/1 -> Saturation1/1
  Sum1/1 -> Sum2/1
  Gain3/1 -> Sum2/2
  Integrator/1 -> Gain1/1, Sum/2
  Integrator2/1 -> "Reference "/1, Gain2/1
  Sum/1 -> Gain/1
  Gain2/1 -> Sum1/2
  "Setpoint "/1 -> Sum/1

== system part2/Reference Model/Setpoint  ==
  nu : Inport
  "eta " : Inport  Port=2
  Constant : Constant  Value=setpoint
  Constant1 : Constant  Value=corner_test
  Constant3 : Constant  Value=corners
  Corner_test : MATLAB Function  TreatAsAtomicUnit=on
  Memory : Memory  InitialCondition=1
  Switch : Switch  Criteria=u2 > Threshold
  "Setpoint " : Outport
  setpoint_change : Outport  Port=2
  wires:
  Constant/1 -> Switch/3
  Switch/1 -> "Setpoint "/1
  Constant1/1 -> Switch/2
  Corner_test/1(setpoint) -> Switch/1
  "eta "/1 -> Corner_test/2(eta)
  nu/1 -> Corner_test/1(nu)
  Constant3/1 -> Corner_test/3(corners)
  Corner_test/3(setpoint_index) -> Memory/1
  Memory/1 -> Corner_test/4("setpoint_index ")
  Corner_test/2(new_setpoint) -> setpoint_change/1

== system part2/Thrust Allocation/Slowly varying angles ==
  u : Inport
  "Freq " : Constant  Value=0.1
  Product : Product
  Product1 : Product
  "Projection " : MATLAB Function  TreatAsAtomicUnit=on
  Sign : Signum
  Sign1 : Signum
  Varying Lowpass Filter : cstblocks/Linear Parameter Varying/Varying Lowpass Filter  N=5
      settings: SourceProductName=Control System Toolbox
  Varying Lowpass Filter1 : cstblocks/Linear Parameter Varying/Varying Lowpass Filter  N=5
      settings: SourceProductName=Control System Toolbox
  Tfs : Outport
  wires:
  "Freq "/1 -> Varying Lowpass Filter/2, Varying Lowpass Filter1/2
  u/1 -> Product/1, "Projection "/1(u)
  Product1/1 -> Tfs/1, "Projection "/2(Tfs)
  Sign/1 -> Product/2, Varying Lowpass Filter1/1
  "Projection "/1(y) -> Sign/1
  Sign1/1 -> Product1/2
  Varying Lowpass Filter1/1 -> Sign1/1
  Varying Lowpass Filter/1 -> Product1/1
  Product/1 -> Varying Lowpass Filter/1

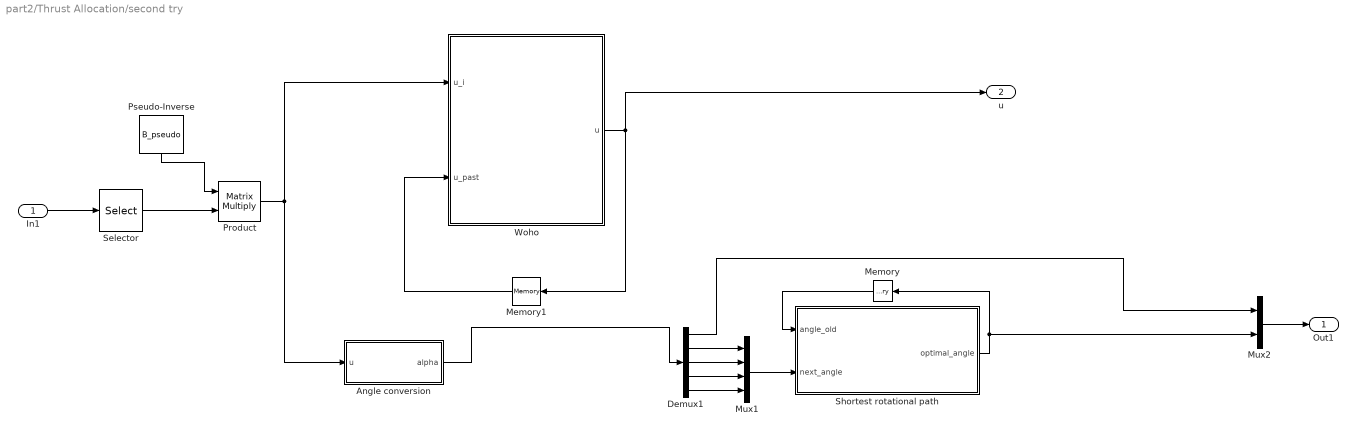
== system part2/Thrust Allocation/second try ==
  In1 : Inport
  Angle conversion : Subsystem
  Demux1 : Demux  Outputs=5
  Memory : Memory
  Memory1 : Memory
  Mux1 : Mux
  Mux2 : Mux  Inputs=2
  Product : Product  Multiplication=Matrix(*)
  Pseudo-Inverse : Constant  Value=B_pseudo
  Selector : Selector  InputPortWidth=6  IndexOptions=Index vector (dialog)  Indices=[1 2 6]  OutputSizes=1
  Shortest rotational path : MATLAB Function  TreatAsAtomicUnit=on
  Woho : MATLAB Function  TreatAsAtomicUnit=on
  Out1 : Outport
  u : Outport  Port=2
  wires:
  Demux1/1 -> Mux2/1
  Demux1/3 -> Mux1/2
  Mux1/1 -> Shortest rotational path/2(next_angle)
  Product/1 -> Angle conversion/1(u), Woho/1(u_i)
  Demux1/4 -> Mux1/3
  Memory/1 -> Shortest rotational path/1(angle_old)
  Woho/1(u) -> u/1, Memory1/1
  Demux1/5 -> Mux1/4
  Shortest rotational path/1(optimal_angle) -> Memory/1, Mux2/2
  Selector/1 -> Product/2
  Memory1/1 -> Woho/2(u_past)
  Pseudo-Inverse/1 -> Product/1
  Demux1/2 -> Mux1/1
  Angle conversion/1(alpha) -> Demux1/1
  In1/1 -> Selector/1
  Mux2/1 -> Out1/1

== system part2/Wind/Wind mean + Gust + Slowly Varying ==
  Gust : Constant  Value=Par_Wind_gust
  Mean angle : Constant  Value=Par_Wind_angle
  Mean velocity : Constant  Value=Par_Wind_V
  Slowly-varying wind : Subsystem  mask(Slowly-varying wind){Par_Wind_sample_time=Par_Wind_sample_time, Par_Wind_speed_T=Par_Wind_speed_T, Par_Wind_angle_T=Par_Wind_angle_T, Par_Wind_speed_noise_pow=Par_Wind_speed_noise_pow, Par_Wind_angle_noise_pow=Par_Wind_angle_noise_pow, Par_Wind_speed_rand_max=Par_Wind_speed_rand_max, Par_Wind_angle_rand_max=Par_Wind_angle_rand_max, Par_Wind_speed_seed=Par_Wind_speed_seed, Par_Wind_angle_seed=Par_Wind_angle_seed}
      mask prompts: Par_Wind_sample_time "Wind sample time [s]"; Par_Wind_speed_T "Wind speed time constant [s]"; Par_Wind_angle_T "Wind angle time constant [s]"; Par_Wind_speed_noise_pow "Wind speed noise power"; Par_Wind_angle_noise_pow "Wind angle noise power"; Par_Wind_speed_rand_max "Wind speed saturation [m/s] (max random variation about mean)"; Par_Wind_angle_rand_max "Wind angle saturation [rad] (max random variation about mean)"; Par_Wind_speed_seed "Wind speed random seed"; Par_Wind_angle_seed "Wind angle random seed"
      mask help:
      | Generate slowly varying wind speed and direction based on random processes.
      |
      | stochastic = 0  gives constant mean wind speed and direction
      | stochastic = 1  gives stochastic mean wind speed and direction
      mask Help:
      | Generate slowly varying wind speed and direction based on random processes.<br>
      | <br>
      | stochastic = 0 gives constant mean wind direction and speed,<br>
      | stochastic = 1 gives stochastic mean wind direction and speed<br>
      | <br>
      | <p>The randomness of the mean speed and angle can be limited by two saturation
      | parameters, which define the maximum random deviation from the mean value.<br>
  Slowlyvar : Constant  Value=Par_Wind_slowlyvar
  Sum : Sum  Inputs=++|  SaturateOnIntegerOverflow=on
  Sum1 : Sum  Inputs=+++  SaturateOnIntegerOverflow=on
  Wind gust : Subsystem  mask(Wind gust){Par_Wind_spectrum_type=Par_Wind_spectrum_type, Par_Wind_phase_seed=Par_Wind_phase_seed, Par_Wind_kappa_H=Par_Wind_kappa_H, Par_Wind_L=Par_Wind_L, Par_Wind_z=Par_Wind_z, Par_Wind_minfreq=Par_Wind_minfreq, Par_Wind_maxfreq=Par_Wind_maxfreq, Par_Wind_nfreq=Par_Wind_nfreq}
      mask prompts: Par_Wind_spectrum_type "Spectrum type"; Par_Wind_phase_seed "Wind gust phase seed"; Par_Wind_kappa_H "Sea surface drag coefficient for Harris wind spectrum (0.0026)"; Par_Wind_L "Scaling length for Harris wind spectrum (1800)"; Par_Wind_z "Height over water surface, for NORSOK spectrum"; Par_Wind_minfreq "Minimum frequency in gust [Hz] (1E-4)"; Par_Wind_maxfreq "Maximum frequency in gust [Hz] (0.1)"; Par_Wind_nfreq "Number of frequency components"
      mask help:
      | Calculate the wind gust according to one of two gust spectra:
      |
      | 1) Harris (based on measurements over land)
      | 2) NORSOK (based on measurements from the North Sea)
      |
      | The gust from the Harris spectrum is not influenced by the heigth over the sea surface, whereas the gust from the NORSOK spectrum is.
  angle : Outport
  speed : Outport  Port=2
  wires:
  Sum1/1 -> speed/1
  Slowly-varying wind/2(speed) -> Sum1/1
  Wind gust/1(Gust) -> Sum1/2
  Sum/1 -> angle/1
  Mean angle/1 -> Sum/1
  Mean velocity/1 -> Sum1/3, Wind gust/1(u10)
  Slowly-varying wind/1(angle) -> Sum/2
  Slowlyvar/1 -> Slowly-varying wind/Enable
  Gust/1 -> Wind gust/Enable

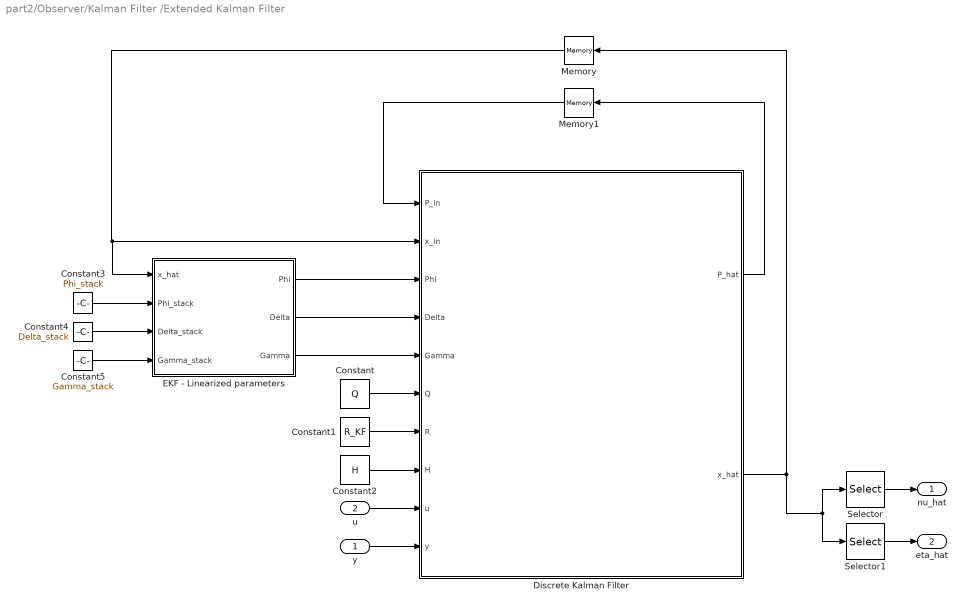
== system part2/Observer/Kalman Filter /Extended Kalman Filter ==
  y : Inport
  u : Inport  Port=2
  Constant : Constant  Value=Q
  Constant1 : Constant  Value=R_KF
  Constant2 : Constant  Value=H
  Constant3 : Constant  Value=Phi_stack
  Constant4 : Constant  Value=Delta_stack
  Constant5 : Constant  Value=Gamma_stack
  Discrete Kalman Filter : MATLAB Function  TreatAsAtomicUnit=on
  EKF - Linearized parameters : MATLAB Function  TreatAsAtomicUnit=on
  Memory : Memory  InitialCondition=zeros(1,15)
  Memory1 : Memory  InitialCondition=eye(15)*0.9
  Selector : Selector  InputPortWidth=15  IndexOptions=Index vector (dialog)  Indices=[13 14 15]  OutputSizes=1
  Selector1 : Selector  InputPortWidth=15  IndexOptions=Index vector (dialog)  Indices=[7 8 9 ]  OutputSizes=1
  nu_hat : Outport
  eta_hat : Outport  Port=2
  wires:
  Discrete Kalman Filter/2(x_hat) -> Selector1/1, Selector/1, Memory/1
  Memory/1 -> EKF - Linearized parameters/1(x_hat), Discrete Kalman Filter/2(x_in)
  y/1 -> Discrete Kalman Filter/10(y)
  Memory1/1 -> Discrete Kalman Filter/1(P_in)
  Selector1/1 -> eta_hat/1
  Selector/1 -> nu_hat/1
  Discrete Kalman Filter/1(P_hat) -> Memory1/1
  u/1 -> Discrete Kalman Filter/9(u)
  Constant5/1 -> EKF - Linearized parameters/4(Gamma_stack)
  Constant3/1 -> EKF - Linearized parameters/2(Phi_stack)
  Constant4/1 -> EKF - Linearized parameters/3(Delta_stack)
  EKF - Linearized parameters/1(Phi) -> Discrete Kalman Filter/3(Phi)
  EKF - Linearized parameters/2(Delta) -> Discrete Kalman Filter/4(Delta)
  EKF - Linearized parameters/3(Gamma) -> Discrete Kalman Filter/5(Gamma)
  Constant2/1 -> Discrete Kalman Filter/8(H)
  Constant1/1 -> Discrete Kalman Filter/7(R)
  Constant/1 -> Discrete Kalman Filter/6(Q)

== system part2/Observer/Non-linear Passive observer/Subsystem ==
  eta : Inport
  tau_est : Inport  Port=2
  " " : Subsystem
  Add : Sum
  Add1 : Sum  Inputs=-+
  Bias estimation : Subsystem
      settings: PortSchema="{\"entries\":[{\"content\":{\"sides\":[{\"content\":{\"connectorIds\":[\"In1\"]},\"type\":\"ConnectorPlacement.EquallySpacedRectSide\",\"uuid\":\"fb609290-747b-4f88-a1dd-5b79b9706ab7\"},{\"content\":{\"connectorIds\":[\"Out1\"],\"side\":\"RIGHT\"},\"type\":\"ConnectorPlacement.EquallySpacedRectSide\",\"uuid\":\"4016d859-7bbf-446e-85bc-2c5f4265ad24\"},{\"content\":{\"connectorIds\":[\"In2\"],\"side\":\"TOP\"},\"type\":\"ConnectorPlacement.EquallySpacedRectSide\",\"uuid\":\"2c9aa93e-b614-4811-8f3b-27afe0a71da6\"}]},\"type\":\"ConnectorPlacement.EquallySpacedConnector\",\"uuid\":\"d56466d4-bbd6-46d5-86ef-c7556ec3bf17\"}],\"packageUris\":[\"http://schema.mathworks.com/mf0/Connector/19700101\"],\"version\":\"1.0\"}"
  K1 : Gain  Gain=K1  Multiplication=Matrix(K*u)
  K2 : Gain  Gain=K2  Multiplication=Matrix(K*u)
  K3 : Gain  Gain=K3  Multiplication=Matrix(K*u)
  K4 : Gain  Gain=K4  Multiplication=Matrix(K*u)
  Vessel dynamics : Subsystem
      settings: PortSchema="{\"entries\":[{\"content\":{\"sides\":[{\"content\":{\"connectorIds\":[\"In1\",\"In2\",\"In3\"]},\"type\":\"ConnectorPlacement.EquallySpacedRectSide\",\"uuid\":\"8c38ab18-b34d-4500-9674-9470dff34018\"},{\"content\":{\"connectorIds\":[\"Out1\"],\"side\":\"RIGHT\"},\"type\":\"ConnectorPlacement.EquallySpacedRectSide\",\"uuid\":\"47c03509-189c-40d1-8765-b41afcba396b\"},{\"content\":{\"connectorIds\":[\"In4\"],\"side\":\"TOP\"},\"type\":\"ConnectorPlacement.EquallySpacedRectSide\",\"uuid\":\"7467cac1-0949-4bd1-891b-658014de3f55\"},{\"content\":{\"connectorIds\":[\"Out2\"],\"side\":\"BOTTOM\"},\"type\":\"ConnectorPlacement.EquallySpacedRectSide\",\"uuid\":\"27535387-606f-426f-80b5-1207c6d5a645\"}]},\"type\":\"ConnectorPlacement.EquallySpacedConnector\",\"uuid\":\"0c384b5b-0f42-40d8-9c98-adb2f646dfa4\"}],\"packageUris\":[\"http://schema.mathworks.com/mf0/Connector/19700101\"],\"version\":\"1.0\"}"
  Wave estimation : Subsystem
  nu_hat : Outport
  eta_hat_total : Outport  Port=2
  wires:
  Wave estimation/1(eta_hat_w) -> Add/1
  " "/1(eta_hat) -> Add/2
  Vessel dynamics/1(out) -> " "/2(input2)
  tau_est/1 -> Vessel dynamics/3(tau_est)
  Bias estimation/1(output) -> Vessel dynamics/4(input3)
  Vessel dynamics/2(nu_hat) -> nu_hat/1
  Add/1 -> Add1/1, eta_hat_total/1
  Add1/1 -> K3/1, K4/1, K2/1, K1/1
  K3/1 -> Bias estimation/1(input)
  K2/1 -> " "/1(input1)
  K1/1 -> Wave estimation/1(input)
  K4/1 -> Vessel dynamics/1(input1)
  eta/1 -> Vessel dynamics/2(eta), Bias estimation/2(eta), Add1/2

== system part2/Thrust Allocation/second try/Angle conversion ==
  u : Inport
  Rotation filtering (not working) : Subsystem
  "atan " : MATLAB Function  TreatAsAtomicUnit=on
  alpha : Outport
  wires:
  "atan "/1(alpha) -> alpha/1
  u/1 -> Rotation filtering (not working)/1(u)
  Rotation filtering (not working)/1(Tfs) -> "atan "/1(Tfs)

== system part2/Wind/Wind mean + Gust + Slowly Varying/Slowly-varying wind ==
  Enable : EnablePort
  Band-Limited White Noise : simulink/Sources/Band-Limited White Noise  Cov=Par_Wind_speed_noise_pow  Ts=Par_Wind_sample_time  seed=Par_Wind_speed_seed
  "Band-Limited White Noise " : simulink/Sources/Band-Limited White Noise  Cov=Par_Wind_angle_noise_pow  Ts=Par_Wind_sample_time  seed=Par_Wind_angle_seed
  Gain : Gain  Gain=1/Par_Wind_speed_T  SaturateOnIntegerOverflow=on  OutDataTypeStr=Inherit: Same as input  ParamDataTypeStr=Inherit: Same as input
  "Gain " : Gain  Gain=1/Par_Wind_angle_T  SaturateOnIntegerOverflow=on  OutDataTypeStr=Inherit: Same as input  ParamDataTypeStr=Inherit: Same as input
  Integrator : Integrator  LimitOutput=on  UpperSaturationLimit=Par_Wind_speed_rand_max  LowerSaturationLimit=-Par_Wind_speed_rand_max
  "Integrator " : Integrator  LimitOutput=on  UpperSaturationLimit=Par_Wind_angle_rand_max  LowerSaturationLimit=-Par_Wind_angle_rand_max
  Sum : Sum  Inputs=|+-  SaturateOnIntegerOverflow=on  InputSameDT=on  OutDataTypeStr=Inherit: Same as first input
  "Sum       " : Sum  Inputs=|+-  SaturateOnIntegerOverflow=on  InputSameDT=on  OutDataTypeStr=Inherit: Same as first input
  angle : Outport  InitialOutput=0
  speed : Outport  Port=2  InitialOutput=0
  wires:
  "Gain "/1 -> "Integrator "/1
  "Sum       "/1 -> "Gain "/1
  "Integrator "/1 -> angle/1, "Sum       "/2
  "Band-Limited White Noise "/1 -> "Sum       "/1
  Gain/1 -> Integrator/1
  Sum/1 -> Gain/1
  Integrator/1 -> speed/1, Sum/2
  Band-Limited White Noise/1 -> Sum/1

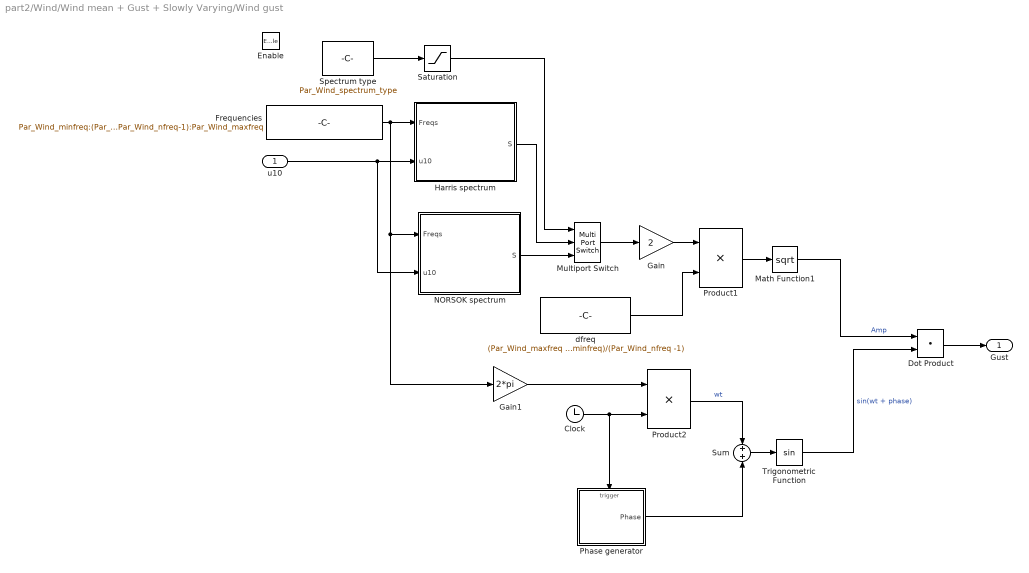
== system part2/Wind/Wind mean + Gust + Slowly Varying/Wind gust ==
  u10 : Inport
  Enable : EnablePort
  Clock : Clock
  Dot Product : DotProduct  InputSameDT=on  OutDataTypeStr=Inherit: Inherit via internal rule
  Frequencies : Constant  Value=Par_Wind_minfreq:(Par_Wind_maxfreq - Par_Wind_minfreq)/(Par_Wind_nfreq-1):Par_Wind_maxfreq
  Gain : Gain  Gain=2  SaturateOnIntegerOverflow=on  OutDataTypeStr=Inherit: Same as input  ParamDataTypeStr=Inherit: Same as input
  Gain1 : Gain  Gain=2*pi  SaturateOnIntegerOverflow=on  OutDataTypeStr=Inherit: Same as input  ParamDataTypeStr=Inherit: Same as input
  Harris spectrum : Subsystem
  Math Function1 : Math  Operator=sqrt  SaturateOnIntegerOverflow=on
  Multiport Switch : MultiPortSwitch  Inputs=2  RndMeth=Nearest  SaturateOnIntegerOverflow=on
  NORSOK spectrum : Subsystem
  Phase generator : Subsystem
  Product1 : Product  SaturateOnIntegerOverflow=on  OutDataTypeStr=Inherit: Same as first input
  Product2 : Product  SaturateOnIntegerOverflow=on  OutDataTypeStr=Inherit: Same as first input
  Saturation : Saturate  UpperLimit=2  LowerLimit=1
  Spectrum type : Constant  Value=Par_Wind_spectrum_type
  Sum : Sum  SaturateOnIntegerOverflow=on
  Trigonometric Function : Trigonometry
  dfreq : Constant  Value=(Par_Wind_maxfreq - Par_Wind_minfreq)/(Par_Wind_nfreq -1)
  Gust : Outport  InitialOutput=0
  wires:
  Dot Product/1 -> Gust/1
  Trigonometric Function/1 -> Dot Product/2  "sin(wt + phase)"
  Math Function1/1 -> Dot Product/1  "Amp"
  Sum/1 -> Trigonometric Function/1
  Phase generator/1(Phase) -> Sum/2
  Product2/1 -> Sum/1  "wt"
  Clock/1 -> Phase generator/Trigger, Product2/2
  Gain1/1 -> Product2/1
  NORSOK spectrum/1(S) -> Multiport Switch/3
  Harris spectrum/1(S) -> Multiport Switch/2
  Spectrum type/1 -> Saturation/1
  Multiport Switch/1 -> Gain/1
  Product1/1 -> Math Function1/1
  dfreq/1 -> Product1/2
  Gain/1 -> Product1/1
  u10/1 -> Harris spectrum/2(u10), NORSOK spectrum/2(u10)
  Frequencies/1 -> Gain1/1, NORSOK spectrum/1(Freqs), Harris spectrum/1(Freqs)
  Saturation/1 -> Multiport Switch/1

== system part2/Observer/Non-linear Passive observer/Subsystem/  ==
  input1 : Inport
  input2 : Inport  Port=2
  Add : Sum
  Integrator : Integrator
  eta_hat : Outport
  wires:
  input2/1 -> Add/2
  Add/1 -> Integrator/1
  Integrator/1 -> eta_hat/1
  input1/1 -> Add/1

== system part2/Observer/Non-linear Passive observer/Subsystem/Bias estimation ==
  input : Inport
  eta : Inport  Port=2
  Integrator : Integrator
  Rot^T : Subsystem
  Subtract : Sum  Inputs=+-
  T^-1 : Gain  Gain=inv(T_b)  Multiplication=Matrix(K*u)
  output : Outport
  wires:
  input/1 -> Subtract/1
  Subtract/1 -> Integrator/1
  Integrator/1 -> Rot^T/2(In2), T^-1/1
  T^-1/1 -> Subtract/2
  eta/1 -> Rot^T/1(eta)
  Rot^T/1(output) -> output/1

== system part2/Observer/Non-linear Passive observer/Subsystem/Vessel dynamics ==
  input1 : Inport
  eta : Inport  Port=2
  tau_est : Inport  Port=3
  input3 : Inport  Port=4
  Add : Sum
  Add1 : Sum  Inputs=++-
  D : Gain  Gain=D  Multiplication=Matrix(K*u)
  Integrator : Integrator
  M^-1 : Gain  Gain=inv(M)  Multiplication=Matrix(K*u)
  Rot : Subsystem
  Rot^T : Subsystem
  out : Outport
  nu_hat : Outport  Port=2
  wires:
  Rot^T/1(output) -> Add/1
  tau_est/1 -> Add/2
  Add/1 -> Add1/2
  input3/1 -> Add1/1
  Add1/1 -> M^-1/1
  M^-1/1 -> Integrator/1
  Integrator/1 -> Rot/2(input1), nu_hat/1, D/1
  Rot/1(output) -> out/1
  D/1 -> Add1/3
  input1/1 -> Rot^T/2(input1)
  eta/1 -> Rot^T/1(eta), Rot/1(eta)

== system part2/Observer/Non-linear Passive observer/Subsystem/Wave estimation ==
  input : Inport
  Add : Sum
  Aw : Gain  Gain=A_w  Multiplication=Matrix(K*u)
  Cw : Gain  Gain=C_w  Multiplication=Matrix(K*u)
  Integrator : Integrator
  eta_hat_w : Outport
  wires:
  input/1 -> Add/1
  Aw/1 -> Add/2
  Add/1 -> Integrator/1
  Integrator/1 -> Aw/1, Cw/1
  Cw/1 -> eta_hat_w/1

== system part2/Thrust Allocation/second try/Angle conversion/Rotation filtering (not working) ==
  u : Inport
  "Freq " : Constant  Value=0.1
  Product : Product
  Product1 : Product
  "Projection " : MATLAB Function  TreatAsAtomicUnit=on
  Sign : Signum
  Sign1 : Signum
  Varying Lowpass Filter : cstblocks/Linear Parameter Varying/Varying Lowpass Filter  N=5
      settings: SourceProductName=Control System Toolbox
  Varying Lowpass Filter1 : cstblocks/Linear Parameter Varying/Varying Lowpass Filter  N=5
      settings: SourceProductName=Control System Toolbox
  Tfs : Outport
  wires:
  "Freq "/1 -> Varying Lowpass Filter/2, Varying Lowpass Filter1/2
  u/1 -> Product/1, "Projection "/1(u)
  Product1/1 -> Tfs/1, "Projection "/2(Tfs)
  Sign/1 -> Product/2, Varying Lowpass Filter1/1
  "Projection "/1(y) -> Sign/1
  Sign1/1 -> Product1/2
  Varying Lowpass Filter1/1 -> Sign1/1
  Varying Lowpass Filter/1 -> Product1/1
  Product/1 -> Varying Lowpass Filter/1

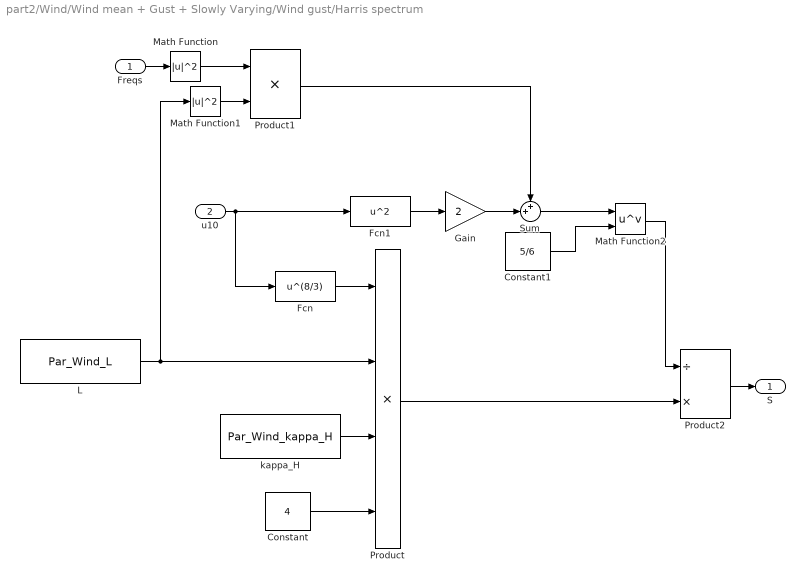
== system part2/Wind/Wind mean + Gust + Slowly Varying/Wind gust/Harris spectrum ==
  Freqs : Inport
  u10 : Inport  Port=2
  Constant : Constant  Value=4
  Constant1 : Constant  Value=5/6
  Fcn : Fcn  Expr=u^(8/3)
  Fcn1 : Fcn  Expr=u^2
  Gain : Gain  Gain=2  SaturateOnIntegerOverflow=on  OutDataTypeStr=Inherit: Same as input  ParamDataTypeStr=Inherit: Same as input
  L : Constant  Value=Par_Wind_L
  Math Function : Math  Operator=magnitude^2  SaturateOnIntegerOverflow=on
  Math Function1 : Math  Operator=magnitude^2  SaturateOnIntegerOverflow=on
  Math Function2 : Math  Operator=pow  SaturateOnIntegerOverflow=on
  Product : Product  Inputs=4  SaturateOnIntegerOverflow=on  OutDataTypeStr=Inherit: Same as first input
  Product1 : Product  SaturateOnIntegerOverflow=on  OutDataTypeStr=Inherit: Same as first input
  Product2 : Product  Inputs=/*  SaturateOnIntegerOverflow=on  OutDataTypeStr=Inherit: Same as first input
  Sum : Sum  Inputs=++|  SaturateOnIntegerOverflow=on
  kappa_H : Constant  Value=Par_Wind_kappa_H
  S : Outport
  wires:
  Product2/1 -> S/1
  Freqs/1 -> Math Function/1
  Product/1 -> Product2/2
  Math Function2/1 -> Product2/1
  Constant1/1 -> Math Function2/2
  Sum/1 -> Math Function2/1
  Product1/1 -> Sum/1
  Math Function1/1 -> Product1/2
  Math Function/1 -> Product1/1
  L/1 -> Math Function1/1, Product/2
  Constant/1 -> Product/4
  Gain/1 -> Sum/2
  Fcn1/1 -> Gain/1
  u10/1 -> Fcn/1, Fcn1/1
  Fcn/1 -> Product/1
  kappa_H/1 -> Product/3

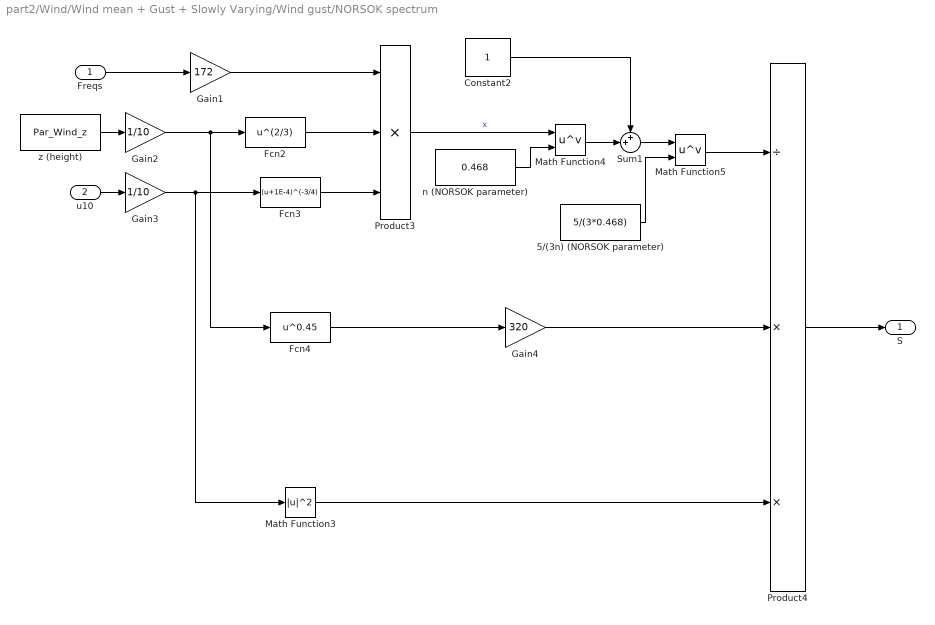
== system part2/Wind/Wind mean + Gust + Slowly Varying/Wind gust/NORSOK spectrum ==
  Freqs : Inport
  u10 : Inport  Port=2
  5/(3n) (NORSOK parameter) : Constant  Value=5/(3*0.468)
  Constant2 : Constant
  Fcn2 : Fcn  Expr=u^(2/3)
  Fcn3 : Fcn  Expr=(u+1E-4)^(-3/4)
  Fcn4 : Fcn  Expr=u^0.45
  Gain1 : Gain  Gain=172  SaturateOnIntegerOverflow=on  OutDataTypeStr=Inherit: Same as input  ParamDataTypeStr=Inherit: Same as input
  Gain2 : Gain  Gain=1/10  SaturateOnIntegerOverflow=on  OutDataTypeStr=Inherit: Same as input  ParamDataTypeStr=Inherit: Same as input
  Gain3 : Gain  Gain=1/10  SaturateOnIntegerOverflow=on  OutDataTypeStr=Inherit: Same as input  ParamDataTypeStr=Inherit: Same as input
  Gain4 : Gain  Gain=320  SaturateOnIntegerOverflow=on  OutDataTypeStr=Inherit: Same as input  ParamDataTypeStr=Inherit: Same as input
  Math Function3 : Math  Operator=magnitude^2  SaturateOnIntegerOverflow=on
  Math Function4 : Math  Operator=pow  SaturateOnIntegerOverflow=on
  Math Function5 : Math  Operator=pow  SaturateOnIntegerOverflow=on
  Product3 : Product  Inputs=3  SaturateOnIntegerOverflow=on  OutDataTypeStr=Inherit: Same as first input
  Product4 : Product  Inputs=/**  SaturateOnIntegerOverflow=on  OutDataTypeStr=Inherit: Same as first input
  Sum1 : Sum  Inputs=++|  SaturateOnIntegerOverflow=on
  n (NORSOK parameter) : Constant  Value=0.468
  z (height) : Constant  Value=Par_Wind_z
  S : Outport
  wires:
  5/(3n) (NORSOK parameter)/1 -> Math Function5/2
  Product4/1 -> S/1
  Gain4/1 -> Product4/2
  Math Function3/1 -> Product4/3
  Fcn4/1 -> Gain4/1
  Math Function5/1 -> Product4/1
  Sum1/1 -> Math Function5/1
  Constant2/1 -> Sum1/1
  Math Function4/1 -> Sum1/2
  n (NORSOK parameter)/1 -> Math Function4/2
  Product3/1 -> Math Function4/1  "x"
  Fcn3/1 -> Product3/3
  Gain3/1 -> Math Function3/1, Fcn3/1
  u10/1 -> Gain3/1
  Fcn2/1 -> Product3/2
  Gain2/1 -> Fcn4/1, Fcn2/1
  z (height)/1 -> Gain2/1
  Gain1/1 -> Product3/1
  Freqs/1 -> Gain1/1

== system part2/Wind/Wind mean + Gust + Slowly Varying/Wind gust/Phase generator ==
  Trigger : TriggerPort  VariantControl=(inherit)
  Random Number : RandomNumber  Variance=3  Seed=Par_Wind_phase_seed*[1:Par_Wind_nfreq]
  "[-inf inf] to [-pi pi]" : marine_gnc/Utilities/Math Operations/[-inf inf] to [-pi pi]
      settings: SourceProductName=MSS GNC
  Phase : Outport
  wires:
  "[-inf inf] to [-pi pi]"/1 -> Phase/1
  Random Number/1 -> "[-inf inf] to [-pi pi]"/1

== system part2/Observer/Non-linear Passive observer/Subsystem/Bias estimation/Rot^T ==
  eta : Inport
  In2 : Inport  Port=2
  Euler angles to rotation matrix : marine_gnc/Models/ Kinematics/Euler angles to rotation matrix
      settings: SourceProductName=MSS GNC
  Matrix Multiply : Product  Multiplication=Matrix(*)
  Transpose : Math  Operator=transpose  SignedPower=off  SaturateOnIntegerOverflow=on
  output : Outport
  wires:
  Euler angles to rotation matrix/1 -> Transpose/1
  eta/1 -> Euler angles to rotation matrix/1
  Transpose/1 -> Matrix Multiply/1
  Matrix Multiply/1 -> output/1
  In2/1 -> Matrix Multiply/2

== system part2/Observer/Non-linear Passive observer/Subsystem/Vessel dynamics/Rot ==
  eta : Inport
  input1 : Inport  Port=2
  Matrix Multiply : Product  Multiplication=Matrix(*)
  euler angles to rotation matrix : marine_gnc/Models/ Kinematics/Euler angles to rotation matrix
      settings: SourceProductName=MSS GNC
  output : Outport
  wires:
  eta/1 -> euler angles to rotation matrix/1
  euler angles to rotation matrix/1 -> Matrix Multiply/1
  Matrix Multiply/1 -> output/1
  input1/1 -> Matrix Multiply/2

== system part2/Observer/Non-linear Passive observer/Subsystem/Vessel dynamics/Rot^T ==
  eta : Inport
  input1 : Inport  Port=2
  Euler angles to rotation matrix : marine_gnc/Models/ Kinematics/Euler angles to rotation matrix
      settings: SourceProductName=MSS GNC
  Matrix Multiply : Product  Multiplication=Matrix(*)
  Transpose : Math  Operator=transpose  SignedPower=off  SaturateOnIntegerOverflow=on
  output : Outport
  wires:
  Euler angles to rotation matrix/1 -> Transpose/1
  eta/1 -> Euler angles to rotation matrix/1
  Transpose/1 -> Matrix Multiply/1
  Matrix Multiply/1 -> output/1
  input1/1 -> Matrix Multiply/2
